simulink library "OBSW"  (Simulink 10.2)
settings: Solver=VariableStepAuto  StartTime=0.0  StopTime=10.0  RelTol=1e-3
undefined symbols (not defined in the file): ACT_MTR_par, OBSW_par
libraries: vrlib x1
settings Model: Creator=dbell44  LastModifiedBy=dbell44

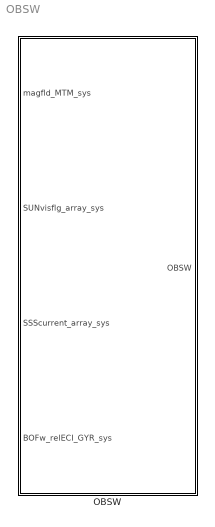
== system OBSW ==
  OBSW : Subsystem

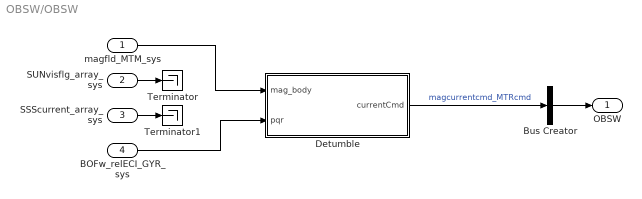
== system OBSW/OBSW ==
  magfld_MTM_sys : Inport
  SUNvisflg_array_sys : Inport  Port=2
  SSScurrent_array_sys : Inport  Port=3
  BOFw_relECI_GYR_sys : Inport  Port=4
  Bus Creator : BusCreator  Inputs=1
  Detumble : Subsystem
  Terminator : Terminator
  Terminator1 : Terminator
  OBSW : Outport
  wires:
  Bus Creator/1 -> OBSW/1
  Detumble/1(currentCmd) -> Bus Creator/1  "magcurrentcmd_MTRcmd"
  magfld_MTM_sys/1 -> Detumble/1(mag_body)
  BOFw_relECI_GYR_sys/1 -> Detumble/2(pqr)
  SUNvisflg_array_sys/1 -> Terminator/1
  SSScurrent_array_sys/1 -> Terminator1/1

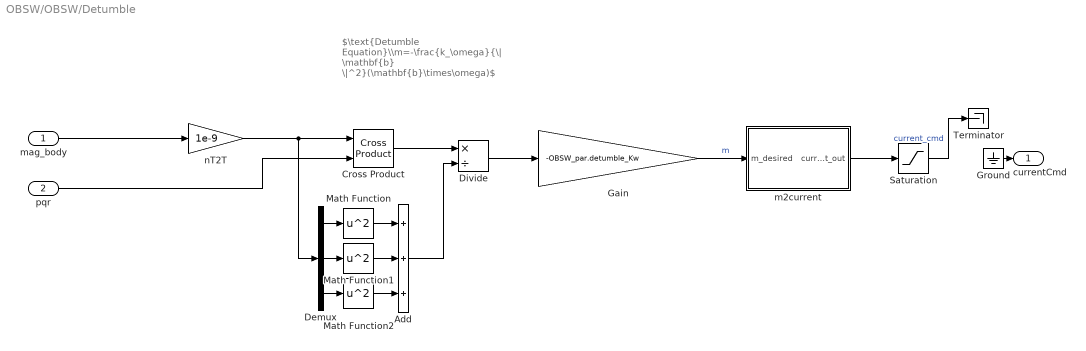
== system OBSW/OBSW/Detumble ==
  note: $\text{Detumble Equation}\\m=-\frac{k_\omega}{\| \mathbf{b} \|^2}(\mathbf{b}\times\omega)$
  mag_body : Inport
  pqr : Inport  Port=2
  Add : Sum  Inputs=+++
  Cross Product : vrlib/Utilities/Cross Product
  Demux : Demux  Outputs=3
  Divide : Product  Inputs=*/
  Gain : Gain  Gain=-OBSW_par.detumble_Kw
  Ground : Ground
  Math Function : Math  Operator=square  SaturateOnIntegerOverflow=on
  Math Function1 : Math  Operator=square  SaturateOnIntegerOverflow=on
  Math Function2 : Math  Operator=square  SaturateOnIntegerOverflow=on
  Saturation : Saturate  UpperLimit=0.1  LowerLimit=0.1  LinearizeAsGain=off
  Terminator : Terminator
  m2current : Subsystem
  nT2T : Gain  Gain=1e-9
  currentCmd : Outport
  wires:
  mag_body/1 -> nT2T/1
  m2current/1(current_out) -> Saturation/1
  Divide/1 -> Gain/1
  Saturation/1 -> Terminator/1  "current_cmd"
  Gain/1 -> m2current/1(m_desired)  "m"
  nT2T/1 -> Demux/1, Cross Product/1
  Add/1 -> Divide/2
  pqr/1 -> Cross Product/2
  Cross Product/1 -> Divide/1
  Demux/1 -> Math Function/1
  Demux/2 -> Math Function1/1
  Demux/3 -> Math Function2/1
  Math Function/1 -> Add/1
  Math Function1/1 -> Add/2
  Math Function2/1 -> Add/3
  Ground/1 -> currentCmd/1

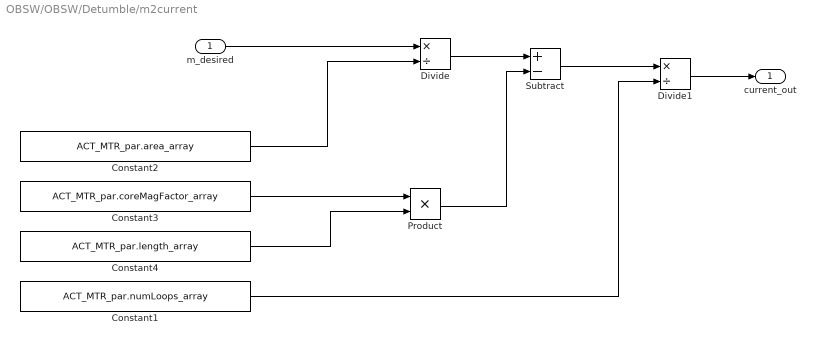
== system OBSW/OBSW/Detumble/m2current ==
  m_desired : Inport
  Constant1 : Constant  Value=ACT_MTR_par.numLoops_array
  Constant2 : Constant  Value=ACT_MTR_par.area_array
  Constant3 : Constant  Value=ACT_MTR_par.coreMagFactor_array
  Constant4 : Constant  Value=ACT_MTR_par.length_array
  Divide : Product  Inputs=*/
  Divide1 : Product  Inputs=*/
  Product : Product
  Subtract : Sum  Inputs=+-
  current_out : Outport
  wires:
  m_desired/1 -> Divide/1
  Constant4/1 -> Product/2
  Product/1 -> Subtract/2
  Divide/1 -> Subtract/1
  Subtract/1 -> Divide1/1
  Constant1/1 -> Divide1/2
  Divide1/1 -> current_out/1
  Constant2/1 -> Divide/2
  Constant3/1 -> Product/1
